simulink model "EnvP_DD"  (R2016b)
settings: configuration reference "CodeGenConfigSet" (kept outside this file)
values from neighbouring files (symbols this model uses):
  EnvP_pPhysRngMax_C = Calibration.Parameter    [init_EnvP_DD.m]
  EnvP_pPhysRngMin_C = Calibration.Parameter    [init_EnvP_DD.m]
  EnvP_pTransf_CUR = Calibration.Parameter    [init_EnvP_DD.m]
  EnvP_pTransf_CURX = Calibration.Parameter    [init_EnvP_DD.m]
  EnvP_tiMaxDefDeb_C = Calibration.Parameter    [init_EnvP_DD.m]
  EnvP_tiMaxOKDeb_C = Calibration.Parameter    [init_EnvP_DD.m]
  EnvP_tiMinDefDeb_C = Calibration.Parameter    [init_EnvP_DD.m]
  EnvP_tiMinOKDeb_C = Calibration.Parameter    [init_EnvP_DD.m]
  EnvP_tiPhysRngHiDefDeb_C = Calibration.Parameter    [init_EnvP_DD.m]
  EnvP_tiPhysRngHiOKDeb_C = Calibration.Parameter    [init_EnvP_DD.m]
  EnvP_tiPhysRngLoDefDeb_C = Calibration.Parameter    [init_EnvP_DD.m]
  EnvP_tiPhysRngLoOKDeb_C = Calibration.Parameter    [init_EnvP_DD.m]
  EnvP_uSRCMax_C = Calibration.Parameter    [init_EnvP_DD.m]
  EnvP_uSRCMin_C = Calibration.Parameter    [init_EnvP_DD.m]
undefined symbols (not defined in the file or in its folder): EnvP_DD_DT
libraries: CXLib x12
settings Model: Creator=lenovo  LastModifiedBy=wangrui
settings ConfigSetRef: SourceLocation=Base Workspace

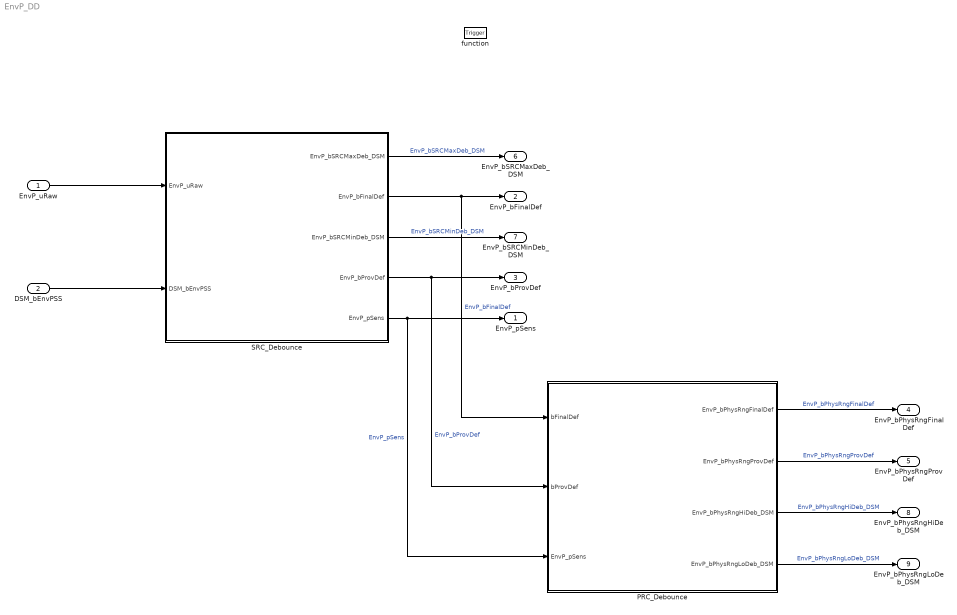
== system EnvP_DD ==
  EnvP_uRaw : Inport  Tag=mv  Description=Sensor signal raw voltage  OutMin=0  OutMax=5000  OutDataTypeStr=Ad_mv
  DSM_bEnvPSS : Inport  Description=state of FId_EnvPSS  Port=2  OutMin=0  OutMax=1  OutDataTypeStr=boolean
  function : TriggerPort  TriggerType=function-call  VariantControl=Variant
  PRC_Debounce : Subsystem
  SRC_Debounce : Subsystem
  EnvP_pSens : Outport  Tag=kPa  Description=Raw physical value  OutMin=0  OutMax=1200  OutDataTypeStr=AirPressure_kPa
  EnvP_bFinalDef : Outport  Description=Environment pressure sensor finally defect flag  Port=2  OutMin=0  OutMax=1  OutDataTypeStr=boolean
  EnvP_bProvDef : Outport  Description=Environment pressure sensor temporary defect flag  Port=3  OutMin=0  OutMax=1  OutDataTypeStr=boolean
  EnvP_bPhysRngFinalDef : Outport  Description=Environment pressure sensor physical range finally defect  Port=4  OutMin=0  OutMax=1  OutDataTypeStr=boolean
  EnvP_bPhysRngProvDef : Outport  Description=Environment pressure sensor physical range temporary defect  Port=5  OutMin=0  OutMax=1  OutDataTypeStr=boolean
  EnvP_bSRCMaxDeb_DSM : Outport  Description=SRC-Max error of Environment pressure sensor  Port=6  OutMin=0  OutMax=1  OutDataTypeStr=boolean
  EnvP_bSRCMinDeb_DSM : Outport  Description=SRC-Min error of Environment pressure sensor  Port=7  OutMin=0  OutMax=1  OutDataTypeStr=boolean
  EnvP_bPhysRngHiDeb_DSM : Outport  Description=Physical-High of Environment pressure sensor  Port=8  OutMin=0  OutMax=1  OutDataTypeStr=boolean
  EnvP_bPhysRngLoDeb_DSM : Outport  Description=Physical-Low of Environment pressure sensor  Port=9  OutMin=0  OutMax=1  OutDataTypeStr=boolean
  wires:
  SRC_Debounce/5(EnvP_pSens) -> EnvP_pSens/1, PRC_Debounce/3(EnvP_pSens)  "EnvP_pSens"
  EnvP_uRaw/1 -> SRC_Debounce/1(EnvP_uRaw)
  DSM_bEnvPSS/1 -> SRC_Debounce/2(DSM_bEnvPSS)
  SRC_Debounce/1(EnvP_bSRCMaxDeb_DSM) -> EnvP_bSRCMaxDeb_DSM/1  "EnvP_bSRCMaxDeb_DSM"
  SRC_Debounce/2(EnvP_bFinalDef) -> EnvP_bFinalDef/1, PRC_Debounce/1(bFinalDef)  "EnvP_bFinalDef"
  SRC_Debounce/3(EnvP_bSRCMinDeb_DSM) -> EnvP_bSRCMinDeb_DSM/1  "EnvP_bSRCMinDeb_DSM"
  SRC_Debounce/4(EnvP_bProvDef) -> EnvP_bProvDef/1, PRC_Debounce/2(bProvDef)  "EnvP_bProvDef"
  PRC_Debounce/1(EnvP_bPhysRngFinalDef) -> EnvP_bPhysRngFinalDef/1  "EnvP_bPhysRngFinalDef"
  PRC_Debounce/2(EnvP_bPhysRngProvDef) -> EnvP_bPhysRngProvDef/1  "EnvP_bPhysRngProvDef"
  PRC_Debounce/3(EnvP_bPhysRngHiDeb_DSM) -> EnvP_bPhysRngHiDeb_DSM/1  "EnvP_bPhysRngHiDeb_DSM"
  PRC_Debounce/4(EnvP_bPhysRngLoDeb_DSM) -> EnvP_bPhysRngLoDeb_DSM/1  "EnvP_bPhysRngLoDeb_DSM"

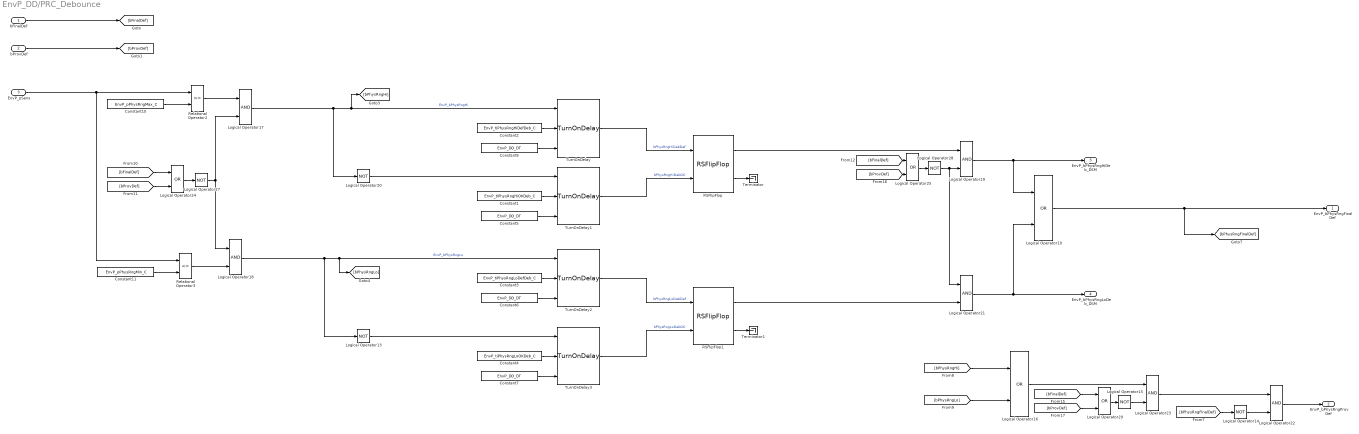
== system EnvP_DD/PRC_Debounce ==
  bFinalDef : Inport
  bProvDef : Inport  Port=2
  EnvP_pSens : Inport  Port=3
  Constant1 : Constant  Value=EnvP_tiPhysRngHiOKDeb_C
  Constant10 : Constant  Value=EnvP_pPhysRngMax_C
  Constant11 : Constant  Value=EnvP_pPhysRngMin_C
  Constant2 : Constant  Value=EnvP_tiPhysRngHiDefDeb_C
  Constant3 : Constant  Value=EnvP_tiPhysRngLoDefDeb_C
  Constant4 : Constant  Value=EnvP_tiPhysRngLoOKDeb_C
  Constant{5..7,9} (4 alike) : Constant  Value=EnvP_DD_DT  OutDataTypeStr=Inherit: Inherit via back propagation
  Logical Operator10 : Logic  Operator=OR  AllPortsSameDT=off  OutDataTypeStr=boolean
  Logical Operator{13..15,20,27..28} (6 alike) : Logic  Operator=NOT  AllPortsSameDT=off  OutDataTypeStr=boolean
  Logical Operator16 : Logic  Operator=OR  AllPortsSameDT=off  OutDataTypeStr=boolean
  Logical Operator{17..19,21..23} (6 alike) : Logic  AllPortsSameDT=off  OutDataTypeStr=boolean
  Logical Operator24 : Logic  RequirementInfo={} %GIDa_74d7f7c9_a87e_44c5_9a2c_7a9ad691ae6c  Operator=OR  OutDataTypeStr=boolean
  Logical Operator25 : Logic  RequirementInfo={} %GIDa_d97bc3d8_1cc0_4861_b4fc_33d8a28a6778  Operator=OR  OutDataTypeStr=boolean
  Logical Operator29 : Logic  RequirementInfo={} %GIDa_ac1768fd_c258_44f0_bfcd_c7b1fef1ab06  Operator=OR  OutDataTypeStr=boolean
  RSFlipFlop : CXLib/RSFlipFlop
  RSFlipFlop1 : CXLib/RSFlipFlop
  Relational Operator2 : RelationalOperator  OutDataTypeStr=boolean  RndMeth=Nearest  InputSameDT=on
  Relational Operator3 : RelationalOperator  Operator=<=  OutDataTypeStr=boolean  RndMeth=Nearest  InputSameDT=on
  Terminator : Terminator
  Terminator1 : Terminator
  TurnOnDelay{,1..3} (4 alike) : CXLib/TurnOnDelay
  EnvP_bPhysRngFinalDef : Outport  OutMin=0  OutMax=1  OutDataTypeStr=boolean
  EnvP_bPhysRngProvDef : Outport  Port=2  OutMin=0  OutMax=1  OutDataTypeStr=boolean
  EnvP_bPhysRngHiDeb_DSM : Outport  Port=3  OutMin=0  OutMax=1  OutDataTypeStr=boolean
  EnvP_bPhysRngLoDeb_DSM : Outport  Port=4  OutMin=0  OutMax=1  OutDataTypeStr=boolean
  wires:
  Logical Operator22/1 -> EnvP_bPhysRngProvDef/1
  Logical Operator23/1 -> Logical Operator22/1
  Logical Operator14/1 -> Logical Operator22/2
  [bPhysRngFinalDef] -> Logical Operator14/1
  Logical Operator29/1 -> Logical Operator15/1
  [bProvDef] -> Logical Operator29/2
  [bFinalDef] -> Logical Operator29/1
  Logical Operator28/1 -> Logical Operator19/2, Logical Operator21/1
  Logical Operator27/1 -> Logical Operator17/2, Logical Operator18/1
  RSFlipFlop1/1 -> Logical Operator21/2
  [bProvDef] -> Logical Operator25/2
  [bFinalDef] -> Logical Operator25/1
  [bProvDef] -> Logical Operator24/2
  [bFinalDef] -> Logical Operator24/1
  Relational Operator3/1 -> Logical Operator18/2
  RSFlipFlop/1 -> Logical Operator19/1
  Logical Operator15/1 -> Logical Operator23/2
  Logical Operator10/1 -> EnvP_bPhysRngFinalDef/1, [bPhysRngFinalDef]
  Logical Operator16/1 -> Logical Operator23/1
  Logical Operator25/1 -> Logical Operator28/1
  Logical Operator24/1 -> Logical Operator27/1
  Relational Operator2/1 -> Logical Operator17/1
  [bPhysRngLo] -> Logical Operator16/2
  [bPhysRngHi] -> Logical Operator16/1
  Logical Operator21/1 -> EnvP_bPhysRngLoDeb_DSM/1, Logical Operator10/2
  Logical Operator19/1 -> EnvP_bPhysRngHiDeb_DSM/1, Logical Operator10/1
  Logical Operator18/1 -> TurnOnDelay2/1, [bPhysRngLo], Logical Operator13/1  "EnvP_bPhysRngLo"
  Constant11/1 -> Relational Operator3/2
  Logical Operator17/1 -> TurnOnDelay/1, [bPhysRngHi], Logical Operator20/1  "EnvP_bPhysRngHi"
  Constant10/1 -> Relational Operator2/2
  Constant7/1 -> TurnOnDelay3/3
  Constant6/1 -> TurnOnDelay2/3
  Constant5/1 -> TurnOnDelay1/3
  Constant9/1 -> TurnOnDelay/3
  TurnOnDelay1/1 -> RSFlipFlop/2  "bPhysRngHiDebOK"
  Constant3/1 -> TurnOnDelay2/2
  Constant1/1 -> TurnOnDelay1/2
  Constant2/1 -> TurnOnDelay/2
  TurnOnDelay/1 -> RSFlipFlop/1  "bPhysRngHiDebDef"
  Logical Operator20/1 -> TurnOnDelay1/1
  TurnOnDelay2/1 -> RSFlipFlop1/1  "bPhysRngLoDebDef"
  Logical Operator13/1 -> TurnOnDelay3/1
  TurnOnDelay3/1 -> RSFlipFlop1/2  "bPhysRngLoDebOK"
  Constant4/1 -> TurnOnDelay3/2
  RSFlipFlop/2 -> Terminator/1
  RSFlipFlop1/2 -> Terminator1/1
  bFinalDef/1 -> [bFinalDef]
  EnvP_pSens/1 -> Relational Operator3/1, Relational Operator2/1
  bProvDef/1 -> [bProvDef]

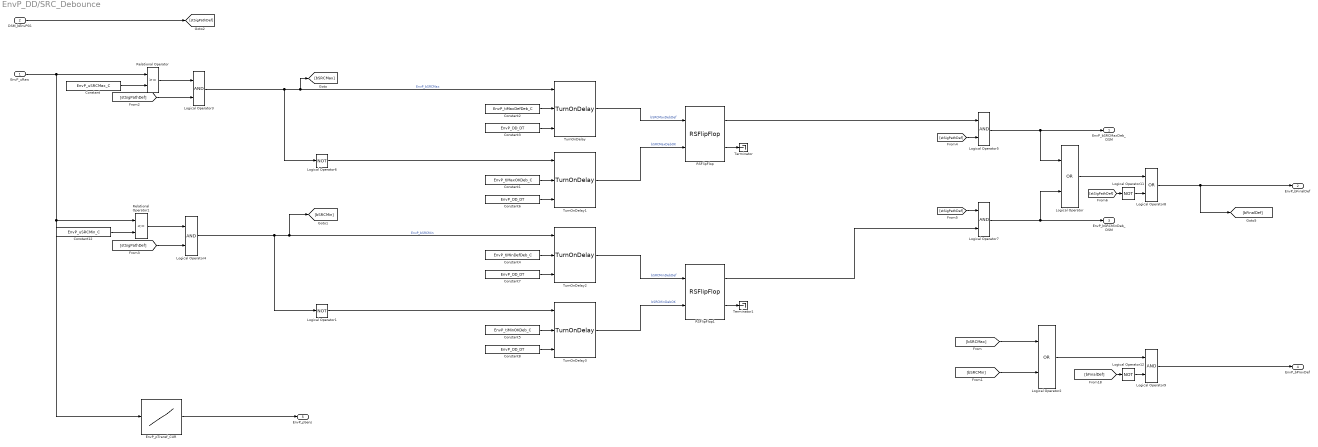
== system EnvP_DD/SRC_Debounce ==
  EnvP_uRaw : Inport  Tag=mv  Description=Sensor signal raw voltage  OutMin=0  OutMax=5000  OutDataTypeStr=Ad_mv
  DSM_bEnvPSS : Inport  Description=state of FId_EnvPSS  Port=2  OutMin=0  OutMax=1  OutDataTypeStr=boolean
  Constant : Constant  Value=EnvP_uSRCMax_C
  Constant1 : Constant  Value=EnvP_tiMaxOKDeb_C
  Constant12 : Constant  Value=EnvP_uSRCMin_C
  Constant2 : Constant  Value=EnvP_tiMaxDefDeb_C
  Constant{3,6..8} (4 alike) : Constant  Value=EnvP_DD_DT  OutDataTypeStr=Inherit: Inherit via back propagation
  Constant4 : Constant  Value=EnvP_tiMinDefDeb_C
  Constant5 : Constant  Value=EnvP_tiMinOKDeb_C
  EnvP_pTransf_CUR : Lookup_n-D  NumberOfTableDimensions=1  BreakpointsForDimension1=EnvP_pTransf_CURX  IndexSearchMethod=Linear search  BeginIndexSearchUsingPreviousIndexResult=on  UseOneInputPortForAllInputData=on  Table=EnvP_pTransf_CUR  ExtrapMethod=Clip  UseLastTableValue=on  InternalRulePriority=Speed  OutDataTypeStr=Inherit: Inherit via back propagation  SaturateOnIntegerOverflow=on
  Logical Operator : Logic  Operator=OR  AllPortsSameDT=off  OutDataTypeStr=boolean
  Logical Operator{1,6,11..12} (4 alike) : Logic  Operator=NOT  AllPortsSameDT=off  OutDataTypeStr=boolean
  Logical Operator2 : Logic  Operator=OR  AllPortsSameDT=off  OutDataTypeStr=boolean
  Logical Operator{3..5,7,9} (5 alike) : Logic  AllPortsSameDT=off  OutDataTypeStr=boolean
  Logical Operator8 : Logic  Operator=OR  AllPortsSameDT=off  OutDataTypeStr=boolean
  RSFlipFlop : CXLib/RSFlipFlop
  RSFlipFlop1 : CXLib/RSFlipFlop
  Relational Operator : RelationalOperator  OutDataTypeStr=boolean  RndMeth=Nearest  InputSameDT=on
  Relational Operator1 : RelationalOperator  Operator=<=  OutDataTypeStr=boolean  RndMeth=Nearest  InputSameDT=on
  Terminator : Terminator
  Terminator1 : Terminator
  TurnOnDelay{,1..3} (4 alike) : CXLib/TurnOnDelay
  EnvP_bSRCMaxDeb_DSM : Outport  OutMin=0  OutMax=1  OutDataTypeStr=boolean
  EnvP_bFinalDef : Outport  Port=2  OutMin=0  OutMax=1  OutDataTypeStr=boolean
  EnvP_bSRCMinDeb_DSM : Outport  Port=3  OutMin=0  OutMax=1  OutDataTypeStr=boolean
  EnvP_bProvDef : Outport  Port=4  OutMin=0  OutMax=1  OutDataTypeStr=boolean
  EnvP_pSens : Outport  Tag=kPa  Description=Raw physical value  Port=5  OutMin=0  OutMax=1200  OutDataTypeStr=AirPressure_kPa
  wires:
  EnvP_pTransf_CUR/1 -> EnvP_pSens/1
  RSFlipFlop1/1 -> Logical Operator7/2
  RSFlipFlop/1 -> Logical Operator5/1
  EnvP_uRaw/1 -> Relational Operator/1, Relational Operator1/1, EnvP_pTransf_CUR/1
  Logical Operator12/1 -> Logical Operator9/2
  Logical Operator11/1 -> Logical Operator8/2
  Logical Operator9/1 -> EnvP_bProvDef/1
  Logical Operator8/1 -> EnvP_bFinalDef/1, [bFinalDef]
  [bFinalDef] -> Logical Operator12/1
  Logical Operator2/1 -> Logical Operator9/1
  [stSigPathDef] -> Logical Operator11/1
  Logical Operator/1 -> Logical Operator8/1
  [stSigPathDef] -> Logical Operator7/1
  [stSigPathDef] -> Logical Operator5/2
  [stSigPathDef] -> Logical Operator4/2
  Relational Operator1/1 -> Logical Operator4/1
  [stSigPathDef] -> Logical Operator3/2
  Relational Operator/1 -> Logical Operator3/1
  DSM_bEnvPSS/1 -> [stSigPathDef]
  [bSRCMin] -> Logical Operator2/2
  [bSRCMax] -> Logical Operator2/1
  Logical Operator7/1 -> EnvP_bSRCMinDeb_DSM/1, Logical Operator/2
  Logical Operator5/1 -> EnvP_bSRCMaxDeb_DSM/1, Logical Operator/1
  Logical Operator4/1 -> Logical Operator1/1, TurnOnDelay2/1, [bSRCMin]  "EnvP_bSRCMin"
  Constant12/1 -> Relational Operator1/2
  Logical Operator3/1 -> Logical Operator6/1, TurnOnDelay/1, [bSRCMax]  "EnvP_bSRCMax"
  Constant/1 -> Relational Operator/2
  Constant8/1 -> TurnOnDelay3/3
  Constant7/1 -> TurnOnDelay2/3
  Constant6/1 -> TurnOnDelay1/3
  Constant3/1 -> TurnOnDelay/3
  RSFlipFlop1/2 -> Terminator1/1
  RSFlipFlop/2 -> Terminator/1
  Constant5/1 -> TurnOnDelay3/2
  TurnOnDelay3/1 -> RSFlipFlop1/2  "bSRCMinDebOK"
  Logical Operator1/1 -> TurnOnDelay3/1
  TurnOnDelay2/1 -> RSFlipFlop1/1  "bSRCMinDebDef"
  Logical Operator6/1 -> TurnOnDelay1/1
  TurnOnDelay/1 -> RSFlipFlop/1  "bSRCMaxDebDef"
  Constant2/1 -> TurnOnDelay/2
  Constant1/1 -> TurnOnDelay1/2
  Constant4/1 -> TurnOnDelay2/2
  TurnOnDelay1/1 -> RSFlipFlop/2  "bSRCMaxDebOK"
